simulink model "CricketBall_Integrate"  (R2017a)
settings: Solver=VariableStepAuto  StartTime=0.0  StopTime=10  RelTol=1e-3
libraries: simulink x1
settings Model: Creator=Prayag  LastModifiedBy=Prayag

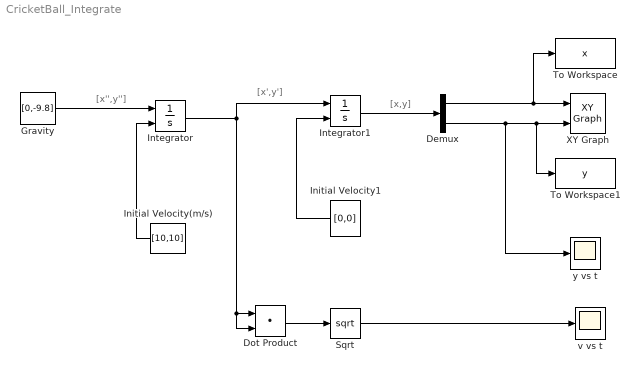
== system CricketBall_Integrate ==
  note: [x'',y'']
  note: [x',y']
  note: [x,y]
  Demux : Demux  Outputs=2
  Dot Product : DotProduct  OutMin=1  InputSameDT=on  OutDataTypeStr=Inherit: Inherit via internal rule
  "Gravity " : Constant  Value=[0,-9.8]
  Initial Velocity(m/s) : Constant  Value=[10,10]
  Initial Velocity1 : Constant  Value=[0,0]
  Integrator : Integrator  InitialConditionSource=external
  Integrator1 : Integrator  InitialConditionSource=external
  Sqrt : Sqrt  SaturateOnIntegerOverflow=on
  To Workspace : ToWorkspace  VariableName=x  SampleTime=-1
  To Workspace1 : ToWorkspace  VariableName=y  SampleTime=-1
  XY Graph : simulink/Sinks/XY Graph  xmin=-1  xmax=25  ymin=0  ymax=15  st=-1
  v vs t : Scope
  y vs t : Scope
  wires:
  Initial Velocity(m/s)/1 -> Integrator/2
  "Gravity "/1 -> Integrator/1
  Integrator/1 -> Integrator1/1, Dot Product/2, Dot Product/1
  Initial Velocity1/1 -> Integrator1/2
  Dot Product/1 -> Sqrt/1
  Sqrt/1 -> v vs t/1
  Integrator1/1 -> Demux/1
  Demux/1 -> To Workspace/1, XY Graph/1
  Demux/2 -> y vs t/1, To Workspace1/1, XY Graph/2
